simulink model "SingleTrackCANoe"  (R2021b)
settings: Solver=ode1  StartTime=0  StopTime=2  FixedStep=1.0000000000000000e-003  RelTol=1e-3
InitFcn:
  | sampleTime = str2double(get_param(bdroot, 'FixedStep'));
undefined symbols (not defined in the file or in its folder): AccPedalPos, BrakePedalPos, BrakeSwitch, DiscIntNeverNeededParam, DYNA4, EngSpd, IgnitionSwitch, InitialGear, InitialSpeed, IntendedEngTrq, LeftIndicator, MainBrakePress, MaxGear, MDL, MinGear, RefAcc, RefLane, RefLatPos, RefPath, RefPathCurv, RefSpd, RefSpdPreview, RefSpdRetrospect, RightIndicator, SteeringWheelAng, SteeringWheelTrq, UserDefinedRefValue, vm_const
libraries: UtilitiesLibrary x62, simulink x18, WheelSystemModules x14, LongitudinalControllerModules x13, LateralControllerModules x7, AnimationBusselectorModules x5, EnvironmentModules x5, BasicEngineControlModules x5, MiscellaneousControlModules x5, Animation3Modules x4, AuxiliariesModules x4, ReducedTireModules x4
(part 21 of 34)

== system SingleTrackCANoe/SimulationModel/Vehicle/Engine/EnginePhysics/InputFromEngineControlUnit ==
  fromEngineControlUnit : Inport
  TDBusSelector : BusSelector  OutputSignals=EngLoadSignal[0_1],EngFuelCutoff[0;1],UpperEngTrqSwitch[0;2],UpperEngTrqLimit[Nm],LowerEngTrqSwitch[0;2],LowerEngTrqLimit[Nm]
  __TDD__EngFuelCutoff[0;1] : Demux  Outputs=1
  __TDD__EngLoadSignal[0_1] : Demux  Outputs=1
  __TDD__LowerEngTrqLimit[Nm] : Demux  Outputs=1
  __TDD__LowerEngTrqSwitch[0;2] : Demux  Outputs=1
  __TDD__UpperEngTrqLimit[Nm] : Demux  Outputs=1
  __TDD__UpperEngTrqSwitch[0;2] : Demux  Outputs=1
  EngLoadSignal[0_1]___UNIQUE_1 : Outport  Description=|  VectorParamsAs1DForOutWhenUnconnected=off
      | <name>EngLoadSignal[0_1]</name>
      | <comment></comment>
  EngFuelCutoff[0;1]___UNIQUE_1 : Outport  Description=|  Port=2  VectorParamsAs1DForOutWhenUnconnected=off
      | <name>EngFuelCutoff[0;1]</name>
      | <comment></comment>
  UpperEngTrqSwitch[0;2]___UNIQUE_1 : Outport  Description=|  Port=3  VectorParamsAs1DForOutWhenUnconnected=off
      | <name>UpperEngTrqSwitch[0;2]</name>
      | <comment></comment>
  UpperEngTrqLimit[Nm]___UNIQUE_1 : Outport  Description=|  Port=4  VectorParamsAs1DForOutWhenUnconnected=off
      | <name>UpperEngTrqLimit[Nm]</name>
      | <comment></comment>
  LowerEngTrqSwitch[0;2]___UNIQUE_1 : Outport  Description=|  Port=5  VectorParamsAs1DForOutWhenUnconnected=off
      | <name>LowerEngTrqSwitch[0;2]</name>
      | <comment></comment>
  LowerEngTrqLimit[Nm]___UNIQUE_1 : Outport  Description=|  Port=6  VectorParamsAs1DForOutWhenUnconnected=off
      | <name>LowerEngTrqLimit[Nm]</name>
      | <comment></comment>
  wires:
  __TDD__LowerEngTrqLimit[Nm]/1 -> LowerEngTrqLimit[Nm]___UNIQUE_1/1  "LowerEngTrqLimit[Nm]"
  __TDD__LowerEngTrqSwitch[0;2]/1 -> LowerEngTrqSwitch[0;2]___UNIQUE_1/1  "LowerEngTrqSwitch[0;2]"
  __TDD__UpperEngTrqLimit[Nm]/1 -> UpperEngTrqLimit[Nm]___UNIQUE_1/1  "UpperEngTrqLimit[Nm]"
  __TDD__UpperEngTrqSwitch[0;2]/1 -> UpperEngTrqSwitch[0;2]___UNIQUE_1/1  "UpperEngTrqSwitch[0;2]"
  __TDD__EngFuelCutoff[0;1]/1 -> EngFuelCutoff[0;1]___UNIQUE_1/1  "EngFuelCutoff[0;1]"
  __TDD__EngLoadSignal[0_1]/1 -> EngLoadSignal[0_1]___UNIQUE_1/1  "EngLoadSignal[0_1]"
  TDBusSelector/6 -> __TDD__LowerEngTrqLimit[Nm]/1  "<LowerEngTrqLimit[Nm]>"
  TDBusSelector/5 -> __TDD__LowerEngTrqSwitch[0;2]/1  "<LowerEngTrqSwitch[0;2]>"
  TDBusSelector/4 -> __TDD__UpperEngTrqLimit[Nm]/1  "<UpperEngTrqLimit[Nm]>"
  TDBusSelector/3 -> __TDD__UpperEngTrqSwitch[0;2]/1  "<UpperEngTrqSwitch[0;2]>"
  TDBusSelector/2 -> __TDD__EngFuelCutoff[0;1]/1  "<EngFuelCutoff[0;1]>"
  TDBusSelector/1 -> __TDD__EngLoadSignal[0_1]/1  "<EngLoadSignal[0_1]>"
  fromEngineControlUnit/1 -> TDBusSelector/1

== system SingleTrackCANoe/SimulationModel/Vehicle/Engine/EnginePhysics/MechanicsOutput ==
  EngTrq[Nm]___UNIQUE_1 : Inport  Description=|  PortDimensions=[1]
      | <name>EngTrq[Nm]</name>
      | <comment></comment>
  MeanEngTrq[Nm]___UNIQUE_1 : Inport  Description=|  Port=2  PortDimensions=[1]
      | <name>MeanEngTrq[Nm]</name>
      | <comment></comment>
  IndicatedTrq[Nm]___UNIQUE_1 : Inport  Description=|  Port=3  PortDimensions=[1]
      | <name>IndicatedTrq[Nm]</name>
      | <comment></comment>
  MeanIndicatedTrq[Nm]___UNIQUE_1 : Inport  Description=|  Port=4  PortDimensions=[1]
      | <name>MeanIndicatedTrq[Nm]</name>
      | <comment></comment>
  MeanEngFrictionTrq[Nm]___UNIQUE_1 : Inport  Description=|  Port=5  PortDimensions=[1]
      | <name>MeanEngFrictionTrq[Nm]</name>
      | <comment></comment>
  MeanEngDragTrq[Nm]___UNIQUE_1 : Inport  Description=|  Port=6  PortDimensions=[1]
      | <name>MeanEngDragTrq[Nm]</name>
      | <comment></comment>
  UnrestrictedEngTrq[Nm]___UNIQUE_1 : Inport  Description=|  Port=7  PortDimensions=[1]
      | <name>UnrestrictedEngTrq[Nm]</name>
      | <comment></comment>
  EngPow[W]___UNIQUE_1 : Inport  Description=|  Port=8  PortDimensions=[1]
      | <name>EngPow[W]</name>
      | <comment></comment>
  EngInrt[kg*m**2]___UNIQUE_1 : Inport  Description=|  Port=9  PortDimensions=[1]
      | <name>EngInrt[kg*m**2]</name>
      | <comment></comment>
  MeanEngMaxTrq[Nm]___UNIQUE_1 : Inport  Description=|  Port=10  PortDimensions=[1]
      | <name>MeanEngMaxTrq[Nm]</name>
      | <comment></comment>
  ThirtyPercentAccPedalEngTrq[Nm]___UNIQUE_1 : Inport  Description=|  Port=11  PortDimensions=[1]
      | <name>ThirtyPercentAccPedalEngTrq[Nm]</name>
      | <comment></comment>
  __SRC__Mechanics.CrankAng[rad] : Constant  Value=0.0  OutDataTypeStr=Inherit: Inherit via back propagation
  __SRC__Mechanics.DerivativeOfEngTrq_wrt_CrankAng[Nm/rad] : Constant  Value=0.0  OutDataTypeStr=Inherit: Inherit via back propagation
  __SRC__Mechanics.DerivativeOfEngTrq_wrt_EngSpd[Nm/(rad/s)] : Constant  Value=0.0  OutDataTypeStr=Inherit: Inherit via back propagation
  __TDD__Mechanics.EngInrt[kg*m**2] : Demux  Outputs=[1]
  __TDD__Mechanics.EngPow[W] : Demux  Outputs=[1]
  __TDD__Mechanics.EngTrq[Nm] : Demux  Outputs=[1]
  __TDD__Mechanics.IndicatedTrq[Nm] : Demux  Outputs=[1]
  __TDD__Mechanics.MeanEngDragTrq[Nm] : Demux  Outputs=[1]
  __TDD__Mechanics.MeanEngFrictionTrq[Nm] : Demux  Outputs=[1]
  __TDD__Mechanics.MeanEngMaxTrq[Nm] : Demux  Outputs=[1]
  __TDD__Mechanics.MeanEngTrq[Nm] : Demux  Outputs=[1]
  __TDD__Mechanics.MeanIndicatedTrq[Nm] : Demux  Outputs=[1]
  __TDD__Mechanics.ThirtyPercentAccPedalEngTrq[Nm] : Demux  Outputs=[1]
  __TDD__Mechanics.UnrestrictedEngTrq[Nm] : Demux  Outputs=[1]
  __TDO__Mechanics : BusCreator  Inputs=14
  Mechanics___UNIQUE_1 : Outport  Description=|  PortDimensions=[14]  VectorParamsAs1DForOutWhenUnconnected=off
      | <name>EngTrq[Nm]</name>
      | <comment></comment>
  wires:
  __TDO__Mechanics/1 -> Mechanics___UNIQUE_1/1  "Mechanics"
  __SRC__Mechanics.DerivativeOfEngTrq_wrt_EngSpd[Nm/(rad/s)]/1 -> __TDO__Mechanics/14  "DerivativeOfEngTrq_wrt_EngSpd[Nm/(rad/s)]"
  __SRC__Mechanics.DerivativeOfEngTrq_wrt_CrankAng[Nm/rad]/1 -> __TDO__Mechanics/13  "DerivativeOfEngTrq_wrt_CrankAng[Nm/rad]"
  __SRC__Mechanics.CrankAng[rad]/1 -> __TDO__Mechanics/12  "CrankAng[rad]"
  __TDD__Mechanics.ThirtyPercentAccPedalEngTrq[Nm]/1 -> __TDO__Mechanics/11  "ThirtyPercentAccPedalEngTrq[Nm]"
  ThirtyPercentAccPedalEngTrq[Nm]___UNIQUE_1/1 -> __TDD__Mechanics.ThirtyPercentAccPedalEngTrq[Nm]/1
  __TDD__Mechanics.MeanEngMaxTrq[Nm]/1 -> __TDO__Mechanics/10  "MeanEngMaxTrq[Nm]"
  MeanEngMaxTrq[Nm]___UNIQUE_1/1 -> __TDD__Mechanics.MeanEngMaxTrq[Nm]/1
  __TDD__Mechanics.EngInrt[kg*m**2]/1 -> __TDO__Mechanics/9  "EngInrt[kg*m**2]"
  EngInrt[kg*m**2]___UNIQUE_1/1 -> __TDD__Mechanics.EngInrt[kg*m**2]/1
  __TDD__Mechanics.EngPow[W]/1 -> __TDO__Mechanics/8  "EngPow[W]"
  EngPow[W]___UNIQUE_1/1 -> __TDD__Mechanics.EngPow[W]/1
  __TDD__Mechanics.UnrestrictedEngTrq[Nm]/1 -> __TDO__Mechanics/7  "UnrestrictedEngTrq[Nm]"
  UnrestrictedEngTrq[Nm]___UNIQUE_1/1 -> __TDD__Mechanics.UnrestrictedEngTrq[Nm]/1
  __TDD__Mechanics.MeanEngDragTrq[Nm]/1 -> __TDO__Mechanics/6  "MeanEngDragTrq[Nm]"
  MeanEngDragTrq[Nm]___UNIQUE_1/1 -> __TDD__Mechanics.MeanEngDragTrq[Nm]/1
  __TDD__Mechanics.MeanEngFrictionTrq[Nm]/1 -> __TDO__Mechanics/5  "MeanEngFrictionTrq[Nm]"
  MeanEngFrictionTrq[Nm]___UNIQUE_1/1 -> __TDD__Mechanics.MeanEngFrictionTrq[Nm]/1
  __TDD__Mechanics.MeanIndicatedTrq[Nm]/1 -> __TDO__Mechanics/4  "MeanIndicatedTrq[Nm]"
  MeanIndicatedTrq[Nm]___UNIQUE_1/1 -> __TDD__Mechanics.MeanIndicatedTrq[Nm]/1
  __TDD__Mechanics.IndicatedTrq[Nm]/1 -> __TDO__Mechanics/3  "IndicatedTrq[Nm]"
  IndicatedTrq[Nm]___UNIQUE_1/1 -> __TDD__Mechanics.IndicatedTrq[Nm]/1
  __TDD__Mechanics.MeanEngTrq[Nm]/1 -> __TDO__Mechanics/2  "MeanEngTrq[Nm]"
  MeanEngTrq[Nm]___UNIQUE_1/1 -> __TDD__Mechanics.MeanEngTrq[Nm]/1
  __TDD__Mechanics.EngTrq[Nm]/1 -> __TDO__Mechanics/1  "EngTrq[Nm]"
  EngTrq[Nm]___UNIQUE_1/1 -> __TDD__Mechanics.EngTrq[Nm]/1

== system SingleTrackCANoe/SimulationModel/Vehicle/Engine/EnginePhysics/ValidityStatus ==
  ValidRangeExceededFlags[-]___UNIQUE_1 : Inport  Description=|  PortDimensions=[1]
      | <name>ValidRangeExceededFlags[-]</name>
      | <comment></comment>
  __TDD__ValidityStatus.ValidRangeExceededFlags[-] : Demux  Outputs=[1]
  __TDO__ValidityStatus : BusCreator  Inputs=1
  ValidityStatus___UNIQUE_1 : Outport  Description=|  PortDimensions=[1]  VectorParamsAs1DForOutWhenUnconnected=off
      | <name>ValidRangeExceededFlags[-]</name>
      | <comment></comment>
  wires:
  __TDO__ValidityStatus/1 -> ValidityStatus___UNIQUE_1/1  "ValidityStatus"
  __TDD__ValidityStatus.ValidRangeExceededFlags[-]/1 -> __TDO__ValidityStatus/1  "ValidRangeExceededFlags[-]"
  ValidRangeExceededFlags[-]___UNIQUE_1/1 -> __TDD__ValidityStatus.ValidRangeExceededFlags[-]/1

== system SingleTrackCANoe/SimulationModel/Vehicle/VehicleRoadInfo/AdditionalRoadElevationAndRoadSlopes/Convert2VehSys ==
  note: RoadSlope(VehSys) = LongRoadSlope(WorldSys)*cos(yaw) + LatRoadSlope(WorldSys)*sin(yaw)
  YawAng[rad] : Inport
  RoadSlopes(WorldSys) : Inport  Port=2
  Demux3 : Demux  Outputs=2
  Product : Product
  Product1 : Product
  Sum : Sum
  Trigonometric Function : Trigonometry
  Trigonometric Function1 : Trigonometry  Operator=cos
  RoadSlopes(VehSys) : Outport  VectorParamsAs1DForOutWhenUnconnected=off
  wires:
  Sum/1 -> RoadSlopes(VehSys)/1
  Product/1 -> Sum/2
  Product1/1 -> Sum/1
  Trigonometric Function1/1 -> Product1/1
  Demux3/2 -> Product/2  "LatRoadSlope"
  Trigonometric Function/1 -> Product/1
  YawAng[rad]/1 -> Trigonometric Function1/1, Trigonometric Function/1
  Demux3/1 -> Product1/2  "LongRoadSlope"
  RoadSlopes(WorldSys)/1 -> Demux3/1

== system SingleTrackCANoe/SimulationModel/Vehicle/WheelSystem/FrontLeftWheelSystem/DynaSystemInfo ==

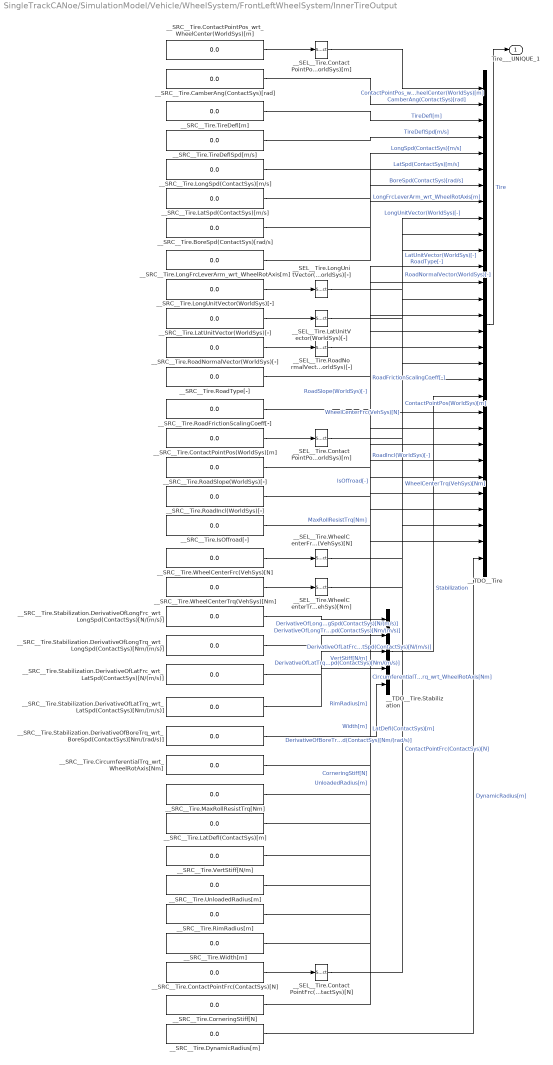
== system SingleTrackCANoe/SimulationModel/Vehicle/WheelSystem/FrontLeftWheelSystem/InnerTireOutput ==
  __SEL__Tire.ContactPointFrc(ContactSys)[N] : Selector  InputPortWidth=1  IndexOptions=Index vector (dialog)  Indices=ones(3, 1)  OutputSizes=1
  __SEL__Tire.ContactPointPos(WorldSys)[m] : Selector  InputPortWidth=1  IndexOptions=Index vector (dialog)  Indices=ones(3, 1)  OutputSizes=1
  __SEL__Tire.ContactPointPos_wrt_WheelCenter(WorldSys)[m] : Selector  InputPortWidth=1  IndexOptions=Index vector (dialog)  Indices=ones(3, 1)  OutputSizes=1
  __SEL__Tire.LatUnitVector(WorldSys)[-] : Selector  InputPortWidth=1  IndexOptions=Index vector (dialog)  Indices=ones(3, 1)  OutputSizes=1
  __SEL__Tire.LongUnitVector(WorldSys)[-] : Selector  InputPortWidth=1  IndexOptions=Index vector (dialog)  Indices=ones(3, 1)  OutputSizes=1
  __SEL__Tire.RoadNormalVector(WorldSys)[-] : Selector  InputPortWidth=1  IndexOptions=Index vector (dialog)  Indices=ones(3, 1)  OutputSizes=1
  __SEL__Tire.WheelCenterFrc(VehSys)[N] : Selector  InputPortWidth=1  IndexOptions=Index vector (dialog)  Indices=ones(3, 1)  OutputSizes=1
  __SEL__Tire.WheelCenterTrq(VehSys)[Nm] : Selector  InputPortWidth=1  IndexOptions=Index vector (dialog)  Indices=ones(3, 1)  OutputSizes=1
  __SRC__Tire.BoreSpd(ContactSys)[rad/s] : Constant  Value=0.0  OutDataTypeStr=Inherit: Inherit via back propagation
  __SRC__Tire.CamberAng(ContactSys)[rad] : Constant  Value=0.0  OutDataTypeStr=Inherit: Inherit via back propagation
  __SRC__Tire.CircumferentialTrq_wrt_WheelRotAxis[Nm] : Constant  Value=0.0  OutDataTypeStr=Inherit: Inherit via back propagation
  __SRC__Tire.ContactPointFrc(ContactSys)[N] : Constant  Value=0.0  OutDataTypeStr=Inherit: Inherit via back propagation
  __SRC__Tire.ContactPointPos(WorldSys)[m] : Constant  Value=0.0  OutDataTypeStr=Inherit: Inherit via back propagation
  __SRC__Tire.ContactPointPos_wrt_WheelCenter(WorldSys)[m] : Constant  Value=0.0  OutDataTypeStr=Inherit: Inherit via back propagation
  __SRC__Tire.CorneringStiff[N] : Constant  Value=0.0  OutDataTypeStr=Inherit: Inherit via back propagation
  __SRC__Tire.DynamicRadius[m] : Constant  Value=0.0  OutDataTypeStr=Inherit: Inherit via back propagation
  __SRC__Tire.IsOffroad[-] : Constant  Value=0.0  OutDataTypeStr=Inherit: Inherit via back propagation
  __SRC__Tire.LatDefl(ContactSys)[m] : Constant  Value=0.0  OutDataTypeStr=Inherit: Inherit via back propagation
  __SRC__Tire.LatSpd(ContactSys)[m/s] : Constant  Value=0.0  OutDataTypeStr=Inherit: Inherit via back propagation
  __SRC__Tire.LatUnitVector(WorldSys)[-] : Constant  Value=0.0  OutDataTypeStr=Inherit: Inherit via back propagation
  __SRC__Tire.LongFrcLeverArm_wrt_WheelRotAxis[m] : Constant  Value=0.0  OutDataTypeStr=Inherit: Inherit via back propagation
  __SRC__Tire.LongSpd(ContactSys)[m/s] : Constant  Value=0.0  OutDataTypeStr=Inherit: Inherit via back propagation
  __SRC__Tire.LongUnitVector(WorldSys)[-] : Constant  Value=0.0  OutDataTypeStr=Inherit: Inherit via back propagation
  __SRC__Tire.MaxRollResistTrq[Nm] : Constant  Value=0.0  OutDataTypeStr=Inherit: Inherit via back propagation
  __SRC__Tire.RimRadius[m] : Constant  Value=0.0  OutDataTypeStr=Inherit: Inherit via back propagation
  __SRC__Tire.RoadFrictionScalingCoeff[-] : Constant  Value=0.0  OutDataTypeStr=Inherit: Inherit via back propagation
  __SRC__Tire.RoadIncl(WorldSys)[-] : Constant  Value=0.0  OutDataTypeStr=Inherit: Inherit via back propagation
  __SRC__Tire.RoadNormalVector(WorldSys)[-] : Constant  Value=0.0  OutDataTypeStr=Inherit: Inherit via back propagation
  __SRC__Tire.RoadSlope(WorldSys)[-] : Constant  Value=0.0  OutDataTypeStr=Inherit: Inherit via back propagation
  __SRC__Tire.RoadType[-] : Constant  Value=0.0  OutDataTypeStr=Inherit: Inherit via back propagation
  __SRC__Tire.Stabilization.DerivativeOfBoreTrq_wrt_BoreSpd(ContactSys)[Nm/(rad/s)] : Constant  Value=0.0  OutDataTypeStr=Inherit: Inherit via back propagation
  __SRC__Tire.Stabilization.DerivativeOfLatFrc_wrt_LatSpd(ContactSys)[N/(m/s)] : Constant  Value=0.0  OutDataTypeStr=Inherit: Inherit via back propagation
  __SRC__Tire.Stabilization.DerivativeOfLatTrq_wrt_LatSpd(ContactSys)[Nm/(m/s)] : Constant  Value=0.0  OutDataTypeStr=Inherit: Inherit via back propagation
  __SRC__Tire.Stabilization.DerivativeOfLongFrc_wrt_LongSpd(ContactSys)[N/(m/s)] : Constant  Value=0.0  OutDataTypeStr=Inherit: Inherit via back propagation
  __SRC__Tire.Stabilization.DerivativeOfLongTrq_wrt_LongSpd(ContactSys)[Nm/(m/s)] : Constant  Value=0.0  OutDataTypeStr=Inherit: Inherit via back propagation
  __SRC__Tire.TireDeflSpd[m/s] : Constant  Value=0.0  OutDataTypeStr=Inherit: Inherit via back propagation
  __SRC__Tire.TireDefl[m] : Constant  Value=0.0  OutDataTypeStr=Inherit: Inherit via back propagation
  __SRC__Tire.UnloadedRadius[m] : Constant  Value=0.0  OutDataTypeStr=Inherit: Inherit via back propagation
  __SRC__Tire.VertStiff[N/m] : Constant  Value=0.0  OutDataTypeStr=Inherit: Inherit via back propagation
  __SRC__Tire.WheelCenterFrc(VehSys)[N] : Constant  Value=0.0  OutDataTypeStr=Inherit: Inherit via back propagation
  __SRC__Tire.WheelCenterTrq(VehSys)[Nm] : Constant  Value=0.0  OutDataTypeStr=Inherit: Inherit via back propagation
  __SRC__Tire.Width[m] : Constant  Value=0.0  OutDataTypeStr=Inherit: Inherit via back propagation
  __TDO__Tire : BusCreator  Inputs=30
  __TDO__Tire.Stabilization : BusCreator  Inputs=5
  Tire___UNIQUE_1 : Outport  Description=|  PortDimensions=[50]  VectorParamsAs1DForOutWhenUnconnected=off
      | <name>ContactPointPos_wrt_WheelCenter(WorldSys)[m]</name>
      | <comment></comment>
  wires:
  __TDO__Tire/1 -> Tire___UNIQUE_1/1  "Tire"
  __SRC__Tire.DynamicRadius[m]/1 -> __TDO__Tire/30  "DynamicRadius[m]"
  __SRC__Tire.CorneringStiff[N]/1 -> __TDO__Tire/29  "CorneringStiff[N]"
  __SEL__Tire.ContactPointFrc(ContactSys)[N]/1 -> __TDO__Tire/28  "ContactPointFrc(ContactSys)[N]"
  __SRC__Tire.Width[m]/1 -> __TDO__Tire/27  "Width[m]"
  __SRC__Tire.RimRadius[m]/1 -> __TDO__Tire/26  "RimRadius[m]"
  __SRC__Tire.UnloadedRadius[m]/1 -> __TDO__Tire/25  "UnloadedRadius[m]"
  __SRC__Tire.VertStiff[N/m]/1 -> __TDO__Tire/24  "VertStiff[N/m]"
  __SRC__Tire.LatDefl(ContactSys)[m]/1 -> __TDO__Tire/23  "LatDefl(ContactSys)[m]"
  __SRC__Tire.MaxRollResistTrq[Nm]/1 -> __TDO__Tire/22  "MaxRollResistTrq[Nm]"
  __SRC__Tire.CircumferentialTrq_wrt_WheelRotAxis[Nm]/1 -> __TDO__Tire/21  "CircumferentialTrq_wrt_WheelRotAxis[Nm]"
  __SRC__Tire.Stabilization.DerivativeOfBoreTrq_wrt_BoreSpd(ContactSys)[Nm/(rad/s)]/1 -> __TDO__Tire.Stabilization/5  "DerivativeOfBoreTrq_wrt_BoreSpd(ContactSys)[Nm/(rad/s)]"
  __SRC__Tire.Stabilization.DerivativeOfLatTrq_wrt_LatSpd(ContactSys)[Nm/(m/s)]/1 -> __TDO__Tire.Stabilization/4  "DerivativeOfLatTrq_wrt_LatSpd(ContactSys)[Nm/(m/s)]"
  __SRC__Tire.Stabilization.DerivativeOfLatFrc_wrt_LatSpd(ContactSys)[N/(m/s)]/1 -> __TDO__Tire.Stabilization/3  "DerivativeOfLatFrc_wrt_LatSpd(ContactSys)[N/(m/s)]"
  __SRC__Tire.Stabilization.DerivativeOfLongTrq_wrt_LongSpd(ContactSys)[Nm/(m/s)]/1 -> __TDO__Tire.Stabilization/2  "DerivativeOfLongTrq_wrt_LongSpd(ContactSys)[Nm/(m/s)]"
  __TDO__Tire.Stabilization/1 -> __TDO__Tire/20  "Stabilization"
  __SRC__Tire.Stabilization.DerivativeOfLongFrc_wrt_LongSpd(ContactSys)[N/(m/s)]/1 -> __TDO__Tire.Stabilization/1  "DerivativeOfLongFrc_wrt_LongSpd(ContactSys)[N/(m/s)]"
  __SEL__Tire.WheelCenterTrq(VehSys)[Nm]/1 -> __TDO__Tire/19  "WheelCenterTrq(VehSys)[Nm]"
  __SEL__Tire.WheelCenterFrc(VehSys)[N]/1 -> __TDO__Tire/18  "WheelCenterFrc(VehSys)[N]"
  __SRC__Tire.IsOffroad[-]/1 -> __TDO__Tire/17  "IsOffroad[-]"
  __SRC__Tire.RoadIncl(WorldSys)[-]/1 -> __TDO__Tire/16  "RoadIncl(WorldSys)[-]"
  __SRC__Tire.RoadSlope(WorldSys)[-]/1 -> __TDO__Tire/15  "RoadSlope(WorldSys)[-]"
  __SEL__Tire.ContactPointPos(WorldSys)[m]/1 -> __TDO__Tire/14  "ContactPointPos(WorldSys)[m]"
  __SRC__Tire.RoadFrictionScalingCoeff[-]/1 -> __TDO__Tire/13  "RoadFrictionScalingCoeff[-]"
  __SRC__Tire.RoadType[-]/1 -> __TDO__Tire/12  "RoadType[-]"
  __SEL__Tire.RoadNormalVector(WorldSys)[-]/1 -> __TDO__Tire/11  "RoadNormalVector(WorldSys)[-]"
  __SEL__Tire.LatUnitVector(WorldSys)[-]/1 -> __TDO__Tire/10  "LatUnitVector(WorldSys)[-]"
  __SEL__Tire.LongUnitVector(WorldSys)[-]/1 -> __TDO__Tire/9  "LongUnitVector(WorldSys)[-]"
  __SRC__Tire.LongFrcLeverArm_wrt_WheelRotAxis[m]/1 -> __TDO__Tire/8  "LongFrcLeverArm_wrt_WheelRotAxis[m]"
  __SRC__Tire.BoreSpd(ContactSys)[rad/s]/1 -> __TDO__Tire/7  "BoreSpd(ContactSys)[rad/s]"
  __SRC__Tire.LatSpd(ContactSys)[m/s]/1 -> __TDO__Tire/6  "LatSpd(ContactSys)[m/s]"
  __SRC__Tire.LongSpd(ContactSys)[m/s]/1 -> __TDO__Tire/5  "LongSpd(ContactSys)[m/s]"
  __SRC__Tire.TireDeflSpd[m/s]/1 -> __TDO__Tire/4  "TireDeflSpd[m/s]"
  __SRC__Tire.TireDefl[m]/1 -> __TDO__Tire/3  "TireDefl[m]"
  __SRC__Tire.CamberAng(ContactSys)[rad]/1 -> __TDO__Tire/2  "CamberAng(ContactSys)[rad]"
  __SEL__Tire.ContactPointPos_wrt_WheelCenter(WorldSys)[m]/1 -> __TDO__Tire/1  "ContactPointPos_wrt_WheelCenter(WorldSys)[m]"
  __SRC__Tire.ContactPointFrc(ContactSys)[N]/1 -> __SEL__Tire.ContactPointFrc(ContactSys)[N]/1
  __SRC__Tire.WheelCenterTrq(VehSys)[Nm]/1 -> __SEL__Tire.WheelCenterTrq(VehSys)[Nm]/1
  __SRC__Tire.WheelCenterFrc(VehSys)[N]/1 -> __SEL__Tire.WheelCenterFrc(VehSys)[N]/1
  __SRC__Tire.ContactPointPos(WorldSys)[m]/1 -> __SEL__Tire.ContactPointPos(WorldSys)[m]/1
  __SRC__Tire.RoadNormalVector(WorldSys)[-]/1 -> __SEL__Tire.RoadNormalVector(WorldSys)[-]/1
  __SRC__Tire.LatUnitVector(WorldSys)[-]/1 -> __SEL__Tire.LatUnitVector(WorldSys)[-]/1
  __SRC__Tire.LongUnitVector(WorldSys)[-]/1 -> __SEL__Tire.LongUnitVector(WorldSys)[-]/1
  __SRC__Tire.ContactPointPos_wrt_WheelCenter(WorldSys)[m]/1 -> __SEL__Tire.ContactPointPos_wrt_WheelCenter(WorldSys)[m]/1
